simulink model "Delta_Omega_Based_Arduino_TCS"  (R2021a)
settings: Solver=FixedStepAuto  StartTime=0.0  StopTime=100  FixedStep=0.001  RelTol=1e-3  EnableMultiTasking=on
values from neighbouring files (symbols this model uses):
  GR = 5    [Model_Data.mat]
  grade = 0    [Model_Data.mat]
  m = 220    [Model_Data.mat]
  r = 0.3059    [Model_Data.mat]
  s2_5_rps = [0 104.6666667 209.3333333 314 418.6666667 523.3333333 628]    [Model_Data.mat]
  s2_5_trq = [70 65 60 50 40 33 27]    [Model_Data.mat]
undefined symbols (not defined in the file or in its folder): conv, h, km, s, T, w
libraries: autolibshared x4, autolibmappedmotor x2, simulink x2, aerolibconvert2 x2, arduinolib x1
(part 1 of 3)
settings Model: SILPILModeSetting=veronly  ExtModeTrigDuration=2  Creator=Raptee - Asusvivo  LastModifiedBy=Raptee - Asusvivo
settings SolverCC: AlgebraicLoopSolver=TrustRegion
settings OptimizationCC: EnhancedBackFolding=on  PassReuseOutputArgsAs=Individual arguments  ZeroExternalMemoryAtStartup=off  ZeroInternalMemoryAtStartup=off  MaxStackSize=64  OptimizeBlockOrder=speed  DifferentSizesBufferReuse=on  OptimizationCustomize=off  EfficientTunableParamExpr=on
settings DebuggingCC: ParameterTunabilityLossMsg=error  SFMachineParentedDataDiag=warning
settings HardwareCC: ProdBitPerPointer=32  ProdBitPerSizeT=32  ProdBitPerPtrDiffT=32  ProdLargestAtomicInteger=Long  ProdLargestAtomicFloat=Double  ProdWordSize=32  ProdHWDeviceType=ARM Compatible->ARM Cortex
settings SFSimCC: MATLABDynamicMemAlloc=off
settings RTWCC: SystemTargetFile=ert.tlc  HardwareBoard=Arduino Due  TemplateMakefile=ert_default_tmf  Toolchain=Arduino ARM  BuildConfiguration=Faster Runs
settings CodeAppCC: ForceParamTrailComments=on  IgnoreCustomStorageClasses=off  OperatorAnnotations=on  SimulinkDataObjDesc=on  SFDataObjDesc=on  InsertBlockDesc=on
settings ERTTargetCC: SupportContinuousTime=on  SupportVariableSizeSignals=on  ExtModeTransport=3  ExtModeStaticAlloc=on  ExtModeStaticAllocSize=24576  ExtModeMexFile=ext_xcp  ExtModeIntrfLevel=Level2 - Open

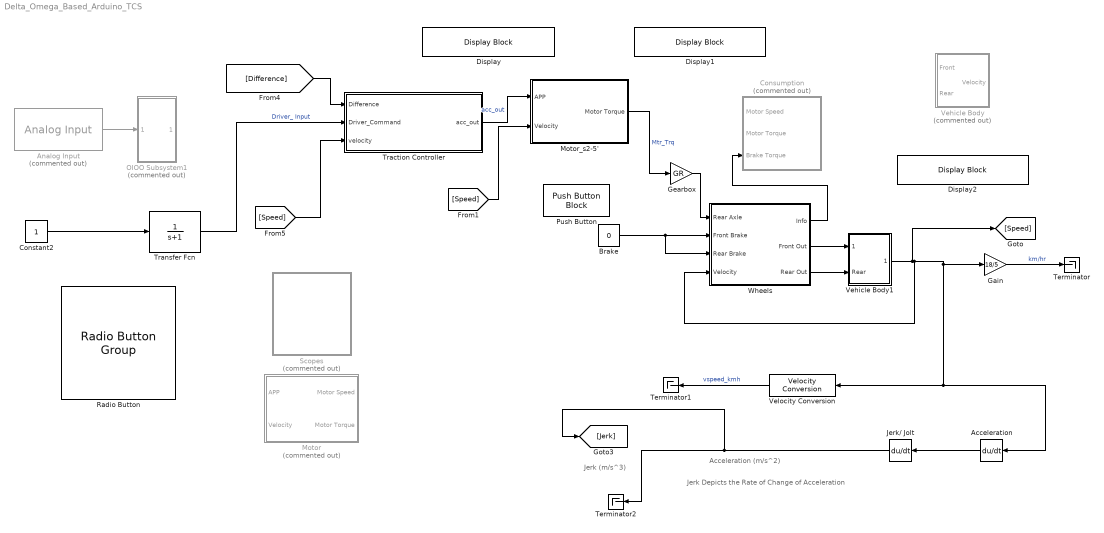
== system Delta_Omega_Based_Arduino_TCS ==
  note: Jerk (m/s^3)
  note: Jerk Depicts the Rate of Change of Acceleration
  note: Acceleration (m/s^2)
  Acceleration : Derivative
  Analog Input : arduinolib/Analog Input  Commented=on  pinNumber=4  ReadResultsOnly=off  ConversionTriggerSource=Software  ExternalTriggerType=uint32( 0 )  OutputDataType=uint16  EnableConversionCompleteNotify=off  EnableOuputStatus=off  SampleTime=-1  blockPlatform=arduino
  Brake : Constant  Value=0
  Constant2 : Constant
  Consumption : Subsystem  Commented=on
  Display : DisplayBlock  LabelPosition=Hide  Format=short  Transparency=1
  Display1 : DisplayBlock  LabelPosition=Hide  Format=short  Transparency=1
  Display2 : DisplayBlock  LabelPosition=Hide  Format=short  Transparency=1
  Gain : Gain  Gain=18/5
  Gearbox : Gain  Gain=GR
  Jerk/ Jolt : Derivative
  "Motor " : Subsystem  Commented=on
  "Motor_s2-5' " : Subsystem
  OIOO Subsystem1 : Subsystem  Commented=on
  Push Button : PushButtonBlock
  Radio Button : RadioButtonGroup  LabelPosition=Hide  SelectedLabel=SPORT  ButtonGroupName=Drive Mode
      settings: Values={{'ECO', 'NORMAL', 'SPORT'}, [1 2 3]}
  Scopes : Subsystem  Commented=on
  Terminator : Terminator
  Terminator1 : Terminator
  Terminator2 : Terminator
  Traction Controller : MATLAB Function  TreatAsAtomicUnit=on
  Transfer Fcn : TransferFcn  Denominator=[1 1]
  Vehicle Body : Subsystem  Commented=on
  Vehicle Body1 : Subsystem
  Velocity Conversion : aerolibconvert2/Velocity Conversion  IU=m/s  OU=km/h
  Wheels : Subsystem
  wires:
  Wheels/3(Rear Out) -> Vehicle Body1/2(Rear)
  Brake/1 -> Wheels/3(Rear Brake), Wheels/2(Front Brake)
  Wheels/1(Info) -> Consumption/3(Brake Torque)
  Gearbox/1 -> Wheels/1(Rear Axle)
  Wheels/2(Front Out) -> Vehicle Body1/1(Front)
  "Motor_s2-5' "/1(Motor Torque) -> Gearbox/1  "Mtr_Trq"
  Gain/1 -> Terminator/1  "km/hr"
  Analog Input/1 -> OIOO Subsystem1/1(Inport)
  Traction Controller/1(acc_out) -> "Motor_s2-5' "/1(APP)  "acc_out"
  Jerk/ Jolt/1 -> Terminator2/1, [Jerk]
  Vehicle Body1/1(Velocity) -> [Speed], Wheels/4(Velocity), Acceleration/1, Velocity Conversion/1, Gain/1
  Acceleration/1 -> Jerk/ Jolt/1
  Velocity Conversion/1 -> Terminator1/1  "vspeed_kmh"
  [Difference] -> Traction Controller/1(Difference)
  [Speed] -> Traction Controller/3(velocity)
  [Speed] -> "Motor_s2-5' "/2(Velocity)
  Constant2/1 -> Transfer Fcn/1
  Transfer Fcn/1 -> Traction Controller/2(Driver_Command)  "Driver_ Input"

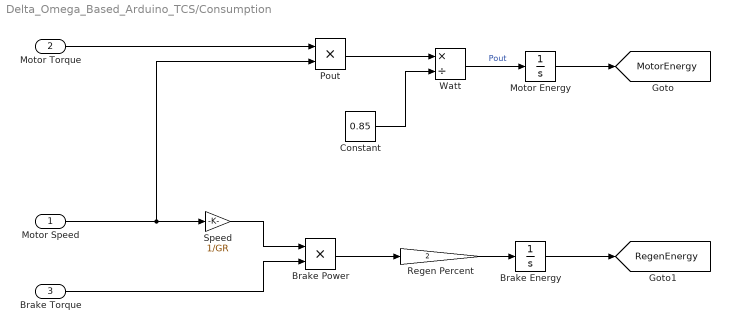
== system Delta_Omega_Based_Arduino_TCS/Consumption ==
  Motor Speed : Inport
  Motor Torque : Inport  Port=2
  Brake Torque : Inport  Port=3
  Brake Energy : Integrator
  Brake Power : Product
  Constant : Constant  Value=0.85
  Motor Energy : Integrator
  Pout : Product
  Regen Percent : Gain  Gain=2
  Speed : Gain  Gain=1/GR
  Watt : Product  Inputs=*/
  tag scope: MotorEnergy=global, RegenEnergy=global
  wires:
  Speed/1 -> Brake Power/1
  Brake Energy/1 -> [RegenEnergy]
  Brake Power/1 -> Regen Percent/1
  Motor Energy/1 -> [MotorEnergy]
  Motor Torque/1 -> Pout/1
  Brake Torque/1 -> Brake Power/2
  Regen Percent/1 -> Brake Energy/1
  Motor Speed/1 -> Speed/1, Pout/2
  Pout/1 -> Watt/1
  Watt/1 -> Motor Energy/1  "Pout"
  Constant/1 -> Watt/2

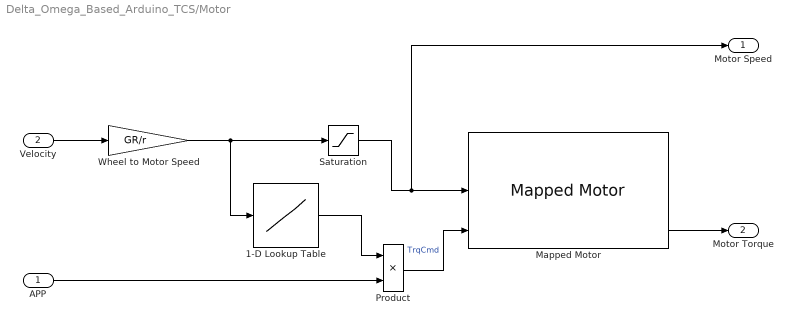
== system Delta_Omega_Based_Arduino_TCS/Motor  ==
  APP : Inport
  Velocity : Inport  Port=2
  1-D Lookup Table : Lookup_n-D  NumberOfTableDimensions=1  BreakpointsForDimension1=w  Table=T  InternalRulePriority=Speed  RndMeth=Simplest  InputSameDT=on
  Mapped Motor : autolibmappedmotor/Mapped Motor  port_config=Speed  param_by=Tabulated torque-speed envelope  w_t=s2_5_rps  T_t=s2_5_trq  torque_max=.1  power_max=30  Tc=0.02  param_loss=Single efficiency measurement  eff=80  w_eff=360  T_eff=29.3  Piron=0  Pbase=0  w_eff_bp=[-8000 -4000 0 4000 8000]  T_eff_bp=[0 0.03 0.06 0.09]  Temp_eff_bp=[233.15 293.15 373.15]  losses_table=[1.49 1.67 2.21 3.10; 0.42 0.69 1.14 2.03; 0.06 0.24 0.78 1.68; 0.42 0.69 1.14 2.03; 1.49 1.67 2.21 3.10]  losses_table_3d=cat(3,1.05*[1.49 1.67 2.21 3.10; 0.42 0.69 1.14 2.03; 0.06 0.24 0.78 1.68; 0.42 0.69 1.14 2.03; 1.49 1.67 2.21 3.10],[1.49 1.67 2.21 3.10; 0.42 0.69 1.14 2.03; 0.06 0.24 0.78 1.68; 0.42 0.69 1.14 2.03; 1.49 1.67 2.21 3.10],1.03*[1.49 1.67 2.21 3.10; 0.42 0.69 1.14 2.03; 0.06 0.24 0.78 1.68; 0.42 0.69 1.14 2.03; 1.49 1.67 2.21 3.10])  efficiency_table=[95 95 95 95; 95 95 95 95; 95 95 95 95; 95 95 95 95; 95 95 95 95]  efficiency_table_3d=cat(3,90*ones(5,4),95*ones(5,4),92*ones(5,4))  J=5e-6  b=1e-5  omega_o=0  T_t_extended=[27 33 40 50 60 65 70 65 60 50 40 33 27]  w_t_extended=[-628 -523.3333333 -418.6666667 -314 -209.3333333 -104.6666667 0 104.6666667 209.3333333 314 418.6666667 523.3333333 628]  KLossIron=0  KLossCopper=3.0717  x_w_eff_vec=[-8000 -4000 0 4000 8000]  x_T_eff_vec=[-0.09 -0.06 -0.03 0 0.03 0.06 0.09]  x_tmp_eff_vec=[233.15 293.15 373.15]  x_losses_mat=[3.1 2.21 1.67 1.49 1.67 2.21 3.1;2.03 1.14 0.69 0.42 0.69 1.14 2.03;1.68 0.78 0.24 0.06 0.24 0.78 1.68;2.03 1.14 0.69 0.42 0.69 1.14 2.03;3.1 2.21 1.67 1.49 1.67 2.21 3.1]  x_losses_mat_3d=cat(3,[3.255 2.3205 1.7535 1.5645 1.7535 2.3205 3.255;2.1315 1.197 0.7245 0.441 0.7245 1.197 2.1315;1.764 0.819 0.252 0.063 0.252 0.819 1.764;2.1315 1.197 0.7245 0.441 0.7245 1.197 2.1315;3.255 2.3205 1.7535 1.5645 1.7535 2.3205 3.255],[3.1 2.21 1.67 1.49 1.67 2.21 3.1;2.03 1.14 0.69 0.42 0.69 1.14 2.03;1.68 0.78 0.24 0.06 0.24 0.78 1.68;2.03 1.14 0.69 0.42 0.69 1.14 2.03;3.1 2.21 1.67 1.49 1.67 2.21 3.1],[3.193 2.2763 1.7201 1.5347 1.7201 2.2763 3.193;2.0909 1.1742 0.7107 0.4326 0.7107 1.1742 2.0909;1.7304 0.8034 0.2472 0.0618 0.2472 0.8034 1.7304;2.0909 1.1742 0.7107 0.4326 0.7107 1.1742 2.0909;3.193 2.2763 1.7201 1.5347 1.7201 2.2763 3.193])  CalLossMapData={}  CalLossWithTempMapData={}  aMode=2  RefBlkName='autolibmappedmotor/Mapped Motor'
      settings: SourceProductBaseCode=PW,DR,MT,UV,VE
  Product : Product
  Saturation : Saturate  UpperLimit=495  LowerLimit=0
  Wheel to Motor Speed : Gain  Gain=GR/r
  Motor Speed : Outport
  Motor Torque : Outport  Port=2
  wires:
  Wheel to Motor Speed/1 -> Saturation/1, 1-D Lookup Table/1
  Product/1 -> Mapped Motor/3  "TrqCmd"
  1-D Lookup Table/1 -> Product/1
  Velocity/1 -> Wheel to Motor Speed/1
  Saturation/1 -> Mapped Motor/2, Motor Speed/1
  Mapped Motor/3 -> Motor Torque/1
  APP/1 -> Product/2

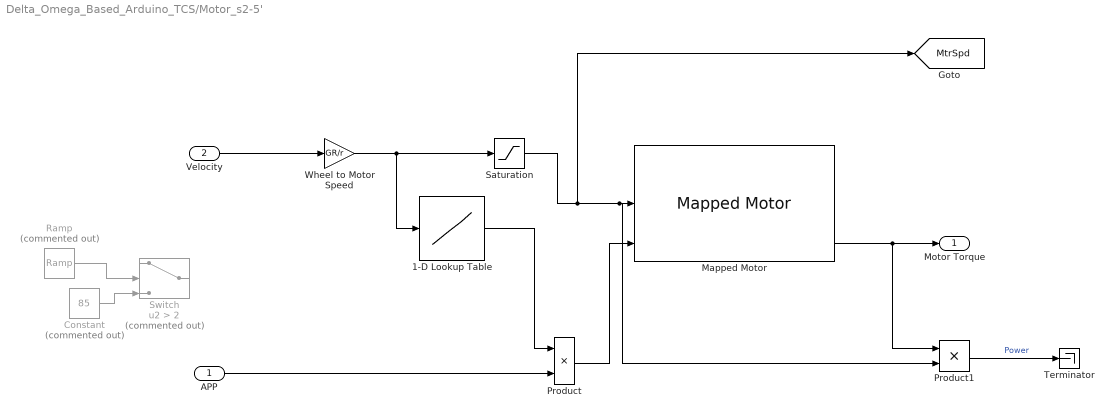
== system Delta_Omega_Based_Arduino_TCS/Motor_s2-5'  ==
  APP : Inport
  Velocity : Inport  Port=2
  1-D Lookup Table : Lookup_n-D  NumberOfTableDimensions=1  BreakpointsForDimension1=s2_5_rps  Table=s2_5_trq  InternalRulePriority=Speed  RndMeth=Simplest  InputSameDT=on
  Constant : Constant  Commented=on  Value=85
  Mapped Motor : autolibmappedmotor/Mapped Motor  port_config=Speed  param_by=Tabulated torque-speed envelope  w_t=s2_5_rps  T_t=s2_5_trq  torque_max=.1  power_max=30  Tc=0.02  param_loss=Single efficiency measurement  eff=80  w_eff=360  T_eff=29.3  Piron=0  Pbase=0  w_eff_bp=[-8000 -4000 0 4000 8000]  T_eff_bp=[0 0.03 0.06 0.09]  Temp_eff_bp=[233.15 293.15 373.15]  losses_table=[1.49 1.67 2.21 3.10; 0.42 0.69 1.14 2.03; 0.06 0.24 0.78 1.68; 0.42 0.69 1.14 2.03; 1.49 1.67 2.21 3.10]  losses_table_3d=cat(3,1.05*[1.49 1.67 2.21 3.10; 0.42 0.69 1.14 2.03; 0.06 0.24 0.78 1.68; 0.42 0.69 1.14 2.03; 1.49 1.67 2.21 3.10],[1.49 1.67 2.21 3.10; 0.42 0.69 1.14 2.03; 0.06 0.24 0.78 1.68; 0.42 0.69 1.14 2.03; 1.49 1.67 2.21 3.10],1.03*[1.49 1.67 2.21 3.10; 0.42 0.69 1.14 2.03; 0.06 0.24 0.78 1.68; 0.42 0.69 1.14 2.03; 1.49 1.67 2.21 3.10])  efficiency_table=[95 95 95 95; 95 95 95 95; 95 95 95 95; 95 95 95 95; 95 95 95 95]  efficiency_table_3d=cat(3,90*ones(5,4),95*ones(5,4),92*ones(5,4))  J=5e-6  b=1e-5  omega_o=0  T_t_extended=[27 33 40 50 60 65 70 65 60 50 40 33 27]  w_t_extended=[-628 -523.3333333 -418.6666667 -314 -209.3333333 -104.6666667 0 104.6666667 209.3333333 314 418.6666667 523.3333333 628]  KLossIron=0  KLossCopper=3.0717  x_w_eff_vec=[-8000 -4000 0 4000 8000]  x_T_eff_vec=[-0.09 -0.06 -0.03 0 0.03 0.06 0.09]  x_tmp_eff_vec=[233.15 293.15 373.15]  x_losses_mat=[3.1 2.21 1.67 1.49 1.67 2.21 3.1;2.03 1.14 0.69 0.42 0.69 1.14 2.03;1.68 0.78 0.24 0.06 0.24 0.78 1.68;2.03 1.14 0.69 0.42 0.69 1.14 2.03;3.1 2.21 1.67 1.49 1.67 2.21 3.1]  x_losses_mat_3d=cat(3,[3.255 2.3205 1.7535 1.5645 1.7535 2.3205 3.255;2.1315 1.197 0.7245 0.441 0.7245 1.197 2.1315;1.764 0.819 0.252 0.063 0.252 0.819 1.764;2.1315 1.197 0.7245 0.441 0.7245 1.197 2.1315;3.255 2.3205 1.7535 1.5645 1.7535 2.3205 3.255],[3.1 2.21 1.67 1.49 1.67 2.21 3.1;2.03 1.14 0.69 0.42 0.69 1.14 2.03;1.68 0.78 0.24 0.06 0.24 0.78 1.68;2.03 1.14 0.69 0.42 0.69 1.14 2.03;3.1 2.21 1.67 1.49 1.67 2.21 3.1],[3.193 2.2763 1.7201 1.5347 1.7201 2.2763 3.193;2.0909 1.1742 0.7107 0.4326 0.7107 1.1742 2.0909;1.7304 0.8034 0.2472 0.0618 0.2472 0.8034 1.7304;2.0909 1.1742 0.7107 0.4326 0.7107 1.1742 2.0909;3.193 2.2763 1.7201 1.5347 1.7201 2.2763 3.193])  CalLossMapData={}  CalLossWithTempMapData={}  aMode=2  RefBlkName='autolibmappedmotor/Mapped Motor'
      settings: SourceProductBaseCode=PW,DR,MT,UV,VE
  Product : Product
  Product1 : Product
  Ramp : simulink/Sources/Ramp  Commented=on  slope=1  start=0  InitialOutput=0
  Saturation : Saturate  UpperLimit=800  LowerLimit=0
  Switch : Switch  Commented=on  Criteria=u2 > Threshold  Threshold=2
  Terminator : Terminator
  Wheel to Motor Speed : Gain  Gain=GR/r
  Motor Torque : Outport
  tag scope: MtrSpd=global
  wires:
  Wheel to Motor Speed/1 -> Saturation/1, 1-D Lookup Table/1
  Product/1 -> Mapped Motor/3
  Velocity/1 -> Wheel to Motor Speed/1
  Saturation/1 -> [MtrSpd], Product1/2, Mapped Motor/2
  Mapped Motor/3 -> Product1/1, Motor Torque/1
  APP/1 -> Product/2
  Ramp/1 -> Switch/2
  Constant/1 -> Switch/3
  1-D Lookup Table/1 -> Product/1
  Product1/1 -> Terminator/1  "Power"

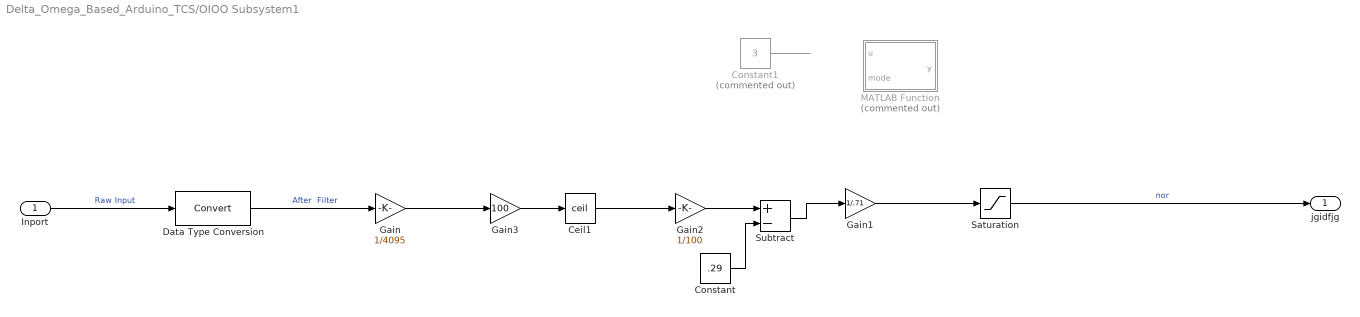
== system Delta_Omega_Based_Arduino_TCS/OIOO Subsystem1 ==
  Inport : Inport
  Ceil1 : Rounding  Operator=ceil
  Constant : Constant  Value=.29
  Constant1 : Constant  Commented=on  Value=3
  Data Type Conversion : DataTypeConversion
  Gain : Gain  Gain=1/4095
  Gain1 : Gain  Gain=1/.71
  Gain2 : Gain  Gain=1/100
  Gain3 : Gain  Gain=100
  MATLAB Function : MATLAB Function  Commented=on  TreatAsAtomicUnit=on
  Saturation : Saturate  UpperLimit=1  LowerLimit=0
  Subtract : Sum  Inputs=+-
  jgidfjg : Outport
  wires:
  Gain/1 -> Gain3/1
  Gain3/1 -> Ceil1/1
  Inport/1 -> Data Type Conversion/1  "Raw Input"
  Gain2/1 -> Subtract/1
  Constant/1 -> Subtract/2
  Subtract/1 -> Gain1/1
  Gain1/1 -> Saturation/1
  Ceil1/1 -> Gain2/1
  Data Type Conversion/1 -> Gain/1  "After  Filter"
  Saturation/1 -> jgidfjg/1  "nor"
  Constant1/1 -> ?

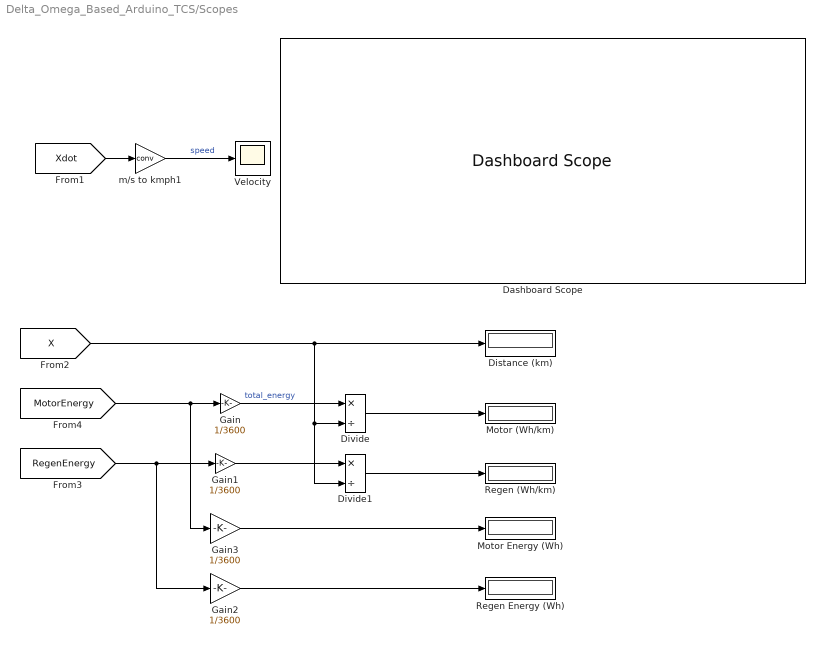
== system Delta_Omega_Based_Arduino_TCS/Scopes ==
  Dashboard Scope : DashboardScope
  Distance (km) : Display
  Divide : Product  Inputs=*/
  Divide1 : Product  Inputs=*/
  Gain{,1..3} (4 alike) : Gain  Gain=1/3600
  Motor (Wh/km) : Display
  Motor Energy (Wh) : Display
  Regen (Wh/km) : Display
  Regen Energy (Wh) : Display
  Velocity : Scope
  m/s to kmph1 : Gain  Gain=conv
  wires:
  [MotorEnergy] -> Gain3/1, Gain/1
  Gain/1 -> Divide/1  "total_energy"
  Gain1/1 -> Divide1/1
  [RegenEnergy] -> Gain2/1, Gain1/1
  Divide/1 -> Motor (Wh/km)/1
  Divide1/1 -> Regen (Wh/km)/1
  m/s to kmph1/1 -> Velocity/1  "speed"
  [X] -> Distance (km)/1, Divide1/2, Divide/2
  [Xdot] -> m/s to kmph1/1
  Gain2/1 -> Regen Energy (Wh)/1
  Gain3/1 -> Motor Energy (Wh)/1

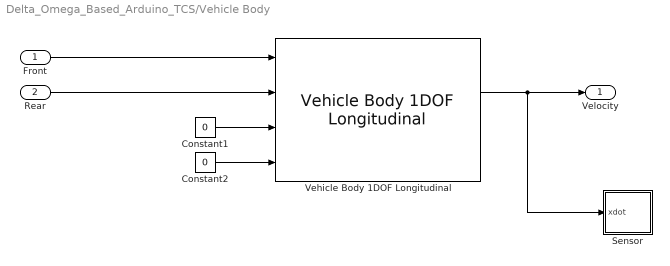
== system Delta_Omega_Based_Arduino_TCS/Vehicle Body ==
  Front : Inport
  Rear : Inport  Port=2
  Constant1 : Constant  Value=0
  Constant2 : Constant  Value=0
  Sensor : Subsystem
  Vehicle Body 1DOF Longitudinal : autolibshared/Vehicle Body 1DOF Longitudinal  VariantControl=SL  extFMode=off  extMMode=off  extTamb=off  wind3D=off  aMode=1  NF=1  NR=1  m=m  a=1.4  b=1.8  h=.35  Cd=.3  Cl=0  Cpm=0  Af=0.9  x_o=0  xdot_o=0  Pabs=101325  T=273  g=9.81
      settings: SourceProductBaseCode=PW,DR,MT,UV,VE
  Velocity : Outport
  wires:
  Rear/1 -> Vehicle Body 1DOF Longitudinal/2
  Constant1/1 -> Vehicle Body 1DOF Longitudinal/3
  Constant2/1 -> Vehicle Body 1DOF Longitudinal/4
  Vehicle Body 1DOF Longitudinal/2 -> Sensor/1(xdot), Velocity/1
  Front/1 -> Vehicle Body 1DOF Longitudinal/1

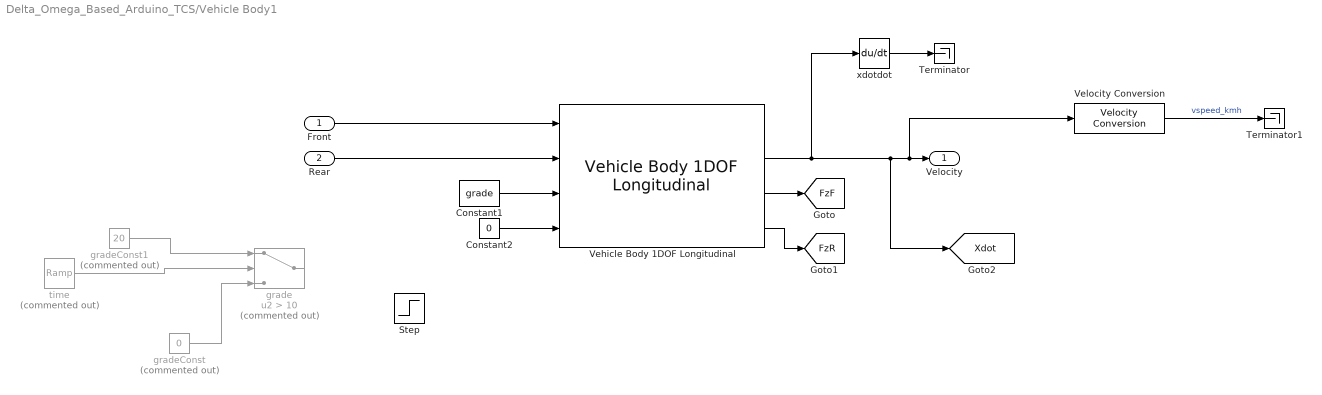
== system Delta_Omega_Based_Arduino_TCS/Vehicle Body1 ==
  Front : Inport
  Rear : Inport  Port=2
  Constant1 : Constant  Value=grade
  Constant2 : Constant  Value=0
  Step : Step  Time=10  After=5.7  SampleTime=0
  Terminator : Terminator
  Terminator1 : Terminator
  Vehicle Body 1DOF Longitudinal : autolibshared/Vehicle Body 1DOF Longitudinal  VariantControl=SL  extFMode=off  extMMode=off  extTamb=off  wind3D=off  aMode=1  NF=1  NR=1  m=m  a=0.738  b=0.706  h=0.597  Cd=Cd  Cl=0  Cpm=0  Af=FrontalArea  x_o=0  xdot_o=0  Pabs=101325  T=273  g=9.81
      settings: SourceProductBaseCode=PW,DR,MT,UV,VE
  Velocity Conversion : aerolibconvert2/Velocity Conversion  IU=m/s  OU=km/h
  grade : Switch  Commented=on  Criteria=u2 > Threshold  Threshold=10
  gradeConst : Constant  Commented=on  Value=0
  gradeConst1 : Constant  Commented=on  Value=20
  time : simulink/Sources/Ramp  Commented=on  slope=1  start=0  InitialOutput=0
  xdotdot : Derivative
  Velocity : Outport
  tag scope: FzF=global, FzR=global, Xdot=global
  wires:
  Rear/1 -> Vehicle Body 1DOF Longitudinal/2
  Constant2/1 -> Vehicle Body 1DOF Longitudinal/4
  Vehicle Body 1DOF Longitudinal/2 -> xdotdot/1, [Xdot], Velocity Conversion/1, Velocity/1
  Front/1 -> Vehicle Body 1DOF Longitudinal/1
  time/1 -> grade/2
  gradeConst1/1 -> grade/1
  gradeConst/1 -> grade/3
  Constant1/1 -> Vehicle Body 1DOF Longitudinal/3
  xdotdot/1 -> Terminator/1
  Vehicle Body 1DOF Longitudinal/3 -> [FzF]
  Vehicle Body 1DOF Longitudinal/4 -> [FzR]
  Velocity Conversion/1 -> Terminator1/1  "vspeed_kmh"
